simulink model "SPI_Thermocouple_2021b"  (R2021b)
settings: Solver=ode3  StartTime=0.0  StopTime=inf  RelTol=1e-3
libraries: arduinolib x4, hdlsllib x1
settings Model: FPTRunName=Active  ExtModeTrigDuration=2  Creator=auw_a  LastModifiedBy=aulwasay
settings SolverCC: AlgebraicLoopSolver=TrustRegion
settings DataIOCC: LimitDataPoints=on  SaveFormat=Array
settings OptimizationCC: ExpressionDepthLimit=2147483647  LifeSpan=Inf  MaxStackSize=64
settings DebuggingCC: UnderspecifiedInitializationDetection=Classic  MergeDetectMultiDrivingBlocksExec=none  FcnCallInpInsideContextMsg=warning  AllowSymbolicDim=off  StateNameClashWarn=warning  SFUnexpectedBacktrackingDiag=warning  SFNoUnconditionalDefaultTransitionDiag=warning  SFExecutionAtInitializationDiag=none  ArithmeticOperatorsInVariantConditions=warning
settings HardwareCC: ProdBitPerInt=16  ProdBitPerPointer=16  ProdBitPerSizeT=16  ProdBitPerPtrDiffT=16  ProdLargestAtomicFloat=None  ProdWordSize=8  ProdHWDeviceType=Atmel->AVR
settings ModelReferenceCC: PropagateSignalLabelsOutOfModel=off
settings SFSimCC: SimUseLocalCustomCode=off  CustomCodeUndefinedFunction=UseInterfaceOnly
settings RTWCC: Description=Embedded Coder  SystemTargetFile=ert.tlc  HardwareBoard=Arduino Uno  TemplateMakefile=ert_default_tmf  GenerateReport=on  RTWVerbose=off  RTWUseLocalCustomCode=off  Toolchain=Arduino AVR  BuildConfiguration=Faster Runs  LaunchReport=on  DLArmComputeVersion=20.02.1
settings CodeAppCC: ForceParamTrailComments=on  OperatorAnnotations=on  StateflowObjectComments=on  MATLABSourceComments=on
settings ERTTargetCC: MultiwordLength=2048  ERTCustomFileBanners=off  SupportContinuousTime=on  SupportNonInlinedSFcns=on  RemoveResetFunc=off  SupportVariableSizeSignals=on  ModelStepFunctionPrototypeControlCompliant=off  ExtModeTransport=3  ExtModeStaticAlloc=on  ExtModeStaticAllocSize=250  ExtModeMexFile=ext_xcp  ExtModeIntrfLevel=Level2 - Open
settings ConfigComp: CovMetricSettings=dw  CovSaveCumulativeToWorkspaceVar=on  CovSaveSingleToWorkspaceVar=on  CovExternalEMLEnable=off  CovSFcnEnable=off

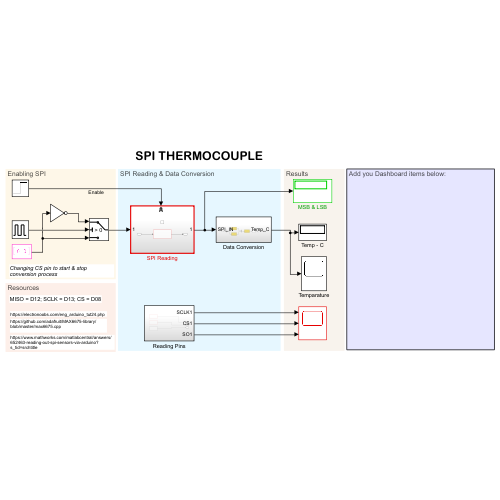
[thumbnail: Simulink's stored preview of the top-level diagram]
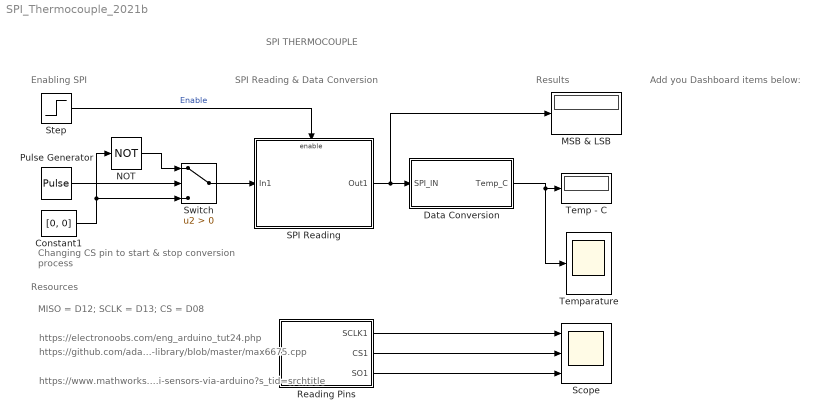
== system SPI_Thermocouple_2021b ==
  note: Add you Dashboard items below:
  note: Changing CS pin to start & stop conversion process
  note: https://www.mathworks.com/matlabcentral/answers/652463-reading-out-spi-sensors-via-arduino?s_tid=srchtitle
  note: https://github.com/adafruit/MAX6675-library/blob/master/max6675.cpp
  note: https://electronoobs.com/eng_arduino_tut24.php
  note: MISO = D12; SCLK = D13; CS = D08
  note: Resources
  note: SPI Reading & Data Conversion
  note: Results
  note: Enabling SPI
  note: SPI THERMOCOUPLE
  Constant1 : Constant  Value=[0, 0]  OutDataTypeStr=uint8
  Data Conversion : Subsystem
  MSB & LSB : Display
  NOT : Logic  Operator=NOT  IconShape=distinctive  AllPortsSameDT=off  OutDataTypeStr=boolean
  Pulse Generator : DiscretePulseGenerator  PulseType=Time based  Period=1  PulseWidth=50
  Reading Pins : Subsystem
  SPI Reading : Subsystem
  Scope : Scope  NumInputPorts=3
  Step : Step  SampleTime=0
  Switch : Switch  Criteria=u2 > Threshold
  Temp - C : Display
  Temparature : Scope
  wires:
  Step/1 -> SPI Reading/Enable  "Enable"
  Constant1/1 -> Switch/3, NOT/1
  Switch/1 -> SPI Reading/1(In1)
  SPI Reading/1(Out1) -> Data Conversion/1(SPI_IN), MSB & LSB/1
  Pulse Generator/1 -> Switch/2
  NOT/1 -> Switch/1
  Data Conversion/1(Temp_C) -> Temparature/1, Temp - C/1
  Reading Pins/1(SCLK1) -> Scope/1
  Reading Pins/2(CS1) -> Scope/2
  Reading Pins/3(SO1) -> Scope/3

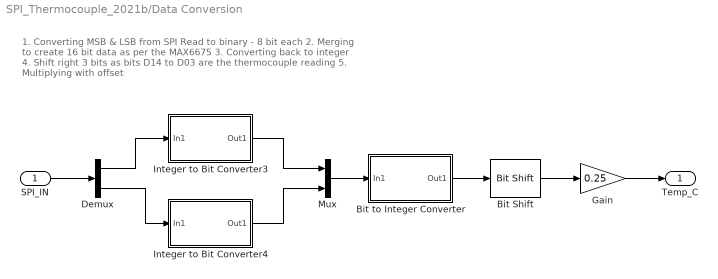
== system SPI_Thermocouple_2021b/Data Conversion ==
  note: 1. Converting MSB & LSB from SPI Read to binary - 8 bit each
      | 2. Merging to create 16 bit data as per the MAX6675
      | 3. Converting back to integer
      | 4. Shift right 3 bits as bits D14 to D03 are the thermocouple reading
      | 5. Multiplying with offset
  SPI_IN : Inport
  Bit Shift : hdlsllib/Logic and Bit Operations/Bit Shift  mode=Shift Right Logical  N=3
  Bit to Integer Converter : Subsystem  Description=Replaced Block  mask(Replaced Block){}
      mask help: This block has been replaced with an empty subsystem because it used functionality that is unavailable in Simulink R2021b.
      mask Display: fprintf('Replaced: %s\n','Bit to Integer Converter')
  Demux : Demux  Outputs=2
  Gain : Gain  Gain=0.25
  Integer to Bit Converter3 : Subsystem  Description=Replaced Block  mask(Replaced Block){}
      mask help: This block has been replaced with an empty subsystem because it used functionality that is unavailable in Simulink R2021b.
      mask Display: fprintf('Replaced: %s\n','Integer to Bit Converter')
  Integer to Bit Converter4 : Subsystem  Description=Replaced Block  mask(Replaced Block){}
      mask help: This block has been replaced with an empty subsystem because it used functionality that is unavailable in Simulink R2021b.
      mask Display: fprintf('Replaced: %s\n','Integer to Bit Converter')
  Mux : Mux  Inputs=2
  Temp_C : Outport
  wires:
  Bit to Integer Converter/1(Out1) -> Bit Shift/1
  Demux/2 -> Integer to Bit Converter4/1(In1)
  Gain/1 -> Temp_C/1
  Demux/1 -> Integer to Bit Converter3/1(In1)
  Integer to Bit Converter3/1(Out1) -> Mux/1
  Bit Shift/1 -> Gain/1
  Mux/1 -> Bit to Integer Converter/1(In1)
  Integer to Bit Converter4/1(Out1) -> Mux/2
  SPI_IN/1 -> Demux/1

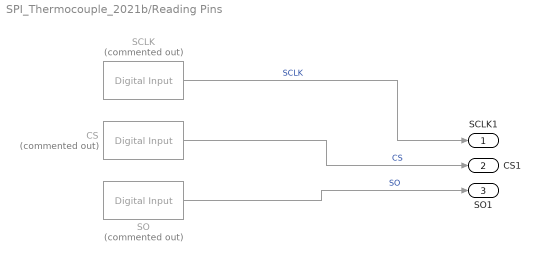
== system SPI_Thermocouple_2021b/Reading Pins ==
  CS : arduinolib/Digital Input  Commented=on  pinNumber=6  mode=Default  Direction=input  SampleTime=0.1  blockPlatform=arduino
  SCLK : arduinolib/Digital Input  Commented=on  pinNumber=5  mode=Default  Direction=input  SampleTime=0.1  blockPlatform=arduino
  SO : arduinolib/Digital Input  Commented=on  pinNumber=7  mode=Default  Direction=input  SampleTime=0.1  blockPlatform=arduino
  SCLK1 : Outport
  CS1 : Outport  Port=2
  SO1 : Outport  Port=3
  wires:
  SCLK/1 -> SCLK1/1  "SCLK"
  CS/1 -> CS1/1  "CS"
  SO/1 -> SO1/1  "SO"

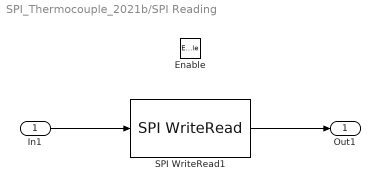
== system SPI_Thermocouple_2021b/SPI Reading ==
  In1 : Inport
  Enable : EnablePort
  SPI WriteRead1 : arduinolib/SPI WriteRead  slaveSelectPin_=8  blockPlatform=arduino
      settings: SourceProductBaseCode=ARDUINO
  Out1 : Outport
  wires:
  In1/1 -> SPI WriteRead1/1
  SPI WriteRead1/1 -> Out1/1

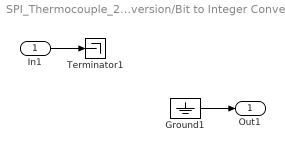
== system SPI_Thermocouple_2021b/Data Conversion/Bit to Integer Converter ==
  In1 : Inport
  Ground1 : Ground
  Terminator1 : Terminator
  Out1 : Outport
  wires:
  Ground1/1 -> Out1/1
  In1/1 -> Terminator1/1

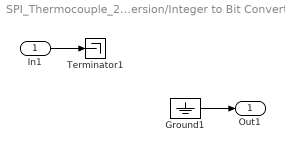
== system SPI_Thermocouple_2021b/Data Conversion/Integer to Bit Converter3 ==
  In1 : Inport
  Ground1 : Ground
  Terminator1 : Terminator
  Out1 : Outport
  wires:
  Ground1/1 -> Out1/1
  In1/1 -> Terminator1/1

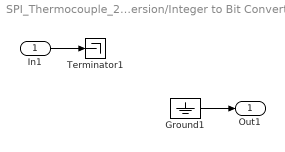
== system SPI_Thermocouple_2021b/Data Conversion/Integer to Bit Converter4 ==
  In1 : Inport
  Ground1 : Ground
  Terminator1 : Terminator
  Out1 : Outport
  wires:
  Ground1/1 -> Out1/1
  In1/1 -> Terminator1/1
